simulink model "PV1000_STM32_767_ZI_state_control"  (R2023a)
settings: Solver=FixedStepAuto  StartTime=0.0  StopTime=inf  FixedStep=0.001  RelTol=1e-3
undefined symbols (not defined in the file): DiscIntNeverNeededParam
libraries: mbedblockslib x17, simulink x14, slpidlib x3, stmnucleolib x2, nucleoutilitieslib x1, etargetslib x1, dspswit3 x1
(part 1 of 2)
settings Model: SimulationMode=external  ExtModeTrigDuration=10  Creator=The MathWorks, Inc.  LastModifiedBy=roehren
settings SolverCC: AlgebraicLoopSolver=TrustRegion  AutoInsertRateTranBlk=on  MaxZcPerStep=1
settings DataIOCC: ReturnWorkspaceOutputs=off
settings OptimizationCC: DefaultParameterBehavior=Inlined  GainParamInheritBuiltInType=on  UseFloatMulNetSlope=on  DefaultUnderspecifiedDataType=single  UseSpecifiedMinMax=on  InlineInvariantSignals=on  ReuseModelBlockBuffer=off  PassReuseOutputArgsAs=Individual arguments  ZeroExternalMemoryAtStartup=off  ZeroInternalMemoryAtStartup=off  NoFixptDivByZeroProtection=on  EfficientFloat2IntCast=on  MaxStackSize=64  OptimizeBlockOrder=speed  EfficientTunableParamExpr=on
settings DebuggingCC: MultiTaskRateTransMsg=warning  ParameterTunabilityLossMsg=error  UnconnectedInputMsg=warning  UnconnectedOutputMsg=warning  UnconnectedLineMsg=warning  ArithmeticOperatorsInVariantConditions=warning
settings HardwareCC: ProdBitPerPointer=32  ProdBitPerSizeT=32  ProdBitPerPtrDiffT=32  ProdLargestAtomicInteger=Long  ProdLargestAtomicFloat=Double  ProdWordSize=32  ProdLongLongMode=on  ProdHWDeviceType=ARM Compatible->ARM Cortex
settings ModelReferenceCC: EnableRefExpFcnMdlSchedulingChecks=on
settings SFSimCC: SimUseLocalCustomCode=off  MATLABDynamicMemAlloc=off
settings RTWCC: Description=Embedded Coder  SystemTargetFile=ert.tlc  HardwareBoard=STM32 Nucleo F767ZI  TemplateMakefile=ert_default_tmf  GenerateReport=on  RTWUseLocalCustomCode=off  Toolchain=GNU Tools for ARM Embedded Processors  BuildConfiguration=Faster Runs  LaunchReport=on  DLArmComputeVersion=19.05
settings CodeAppCC: ForceParamTrailComments=on  OperatorAnnotations=on  StateflowObjectComments=on  MATLABSourceComments=on
settings ERTTargetCC: CodeReplacementLibrary=ARM Cortex-M (Optimized)  MultiwordLength=2048  CombineSignalStateStructs=on  ERTCustomFileBanners=off  SupportNonFinite=off  SupportContinuousTime=on  RemoveResetFunc=off  ModelStepFunctionPrototypeControlCompliant=off  ExtModeTransport=3  ExtModeStaticAlloc=on  ExtModeStaticAllocSize=2000  ExtModeMexFile=ext_xcp  ExtModeIntrfLevel=Level2 - Open
settings ConfigComp: CovMetricSettings=dsw  CovSaveCumulativeToWorkspaceVar=on  CovSaveSingleToWorkspaceVar=on  CovExternalEMLEnable=off

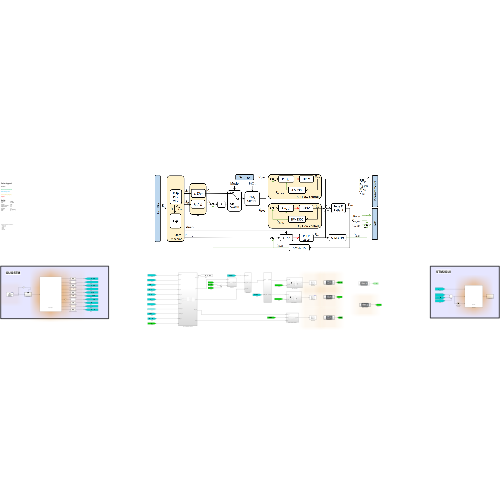
[thumbnail: Simulink's stored preview of the top-level diagram]
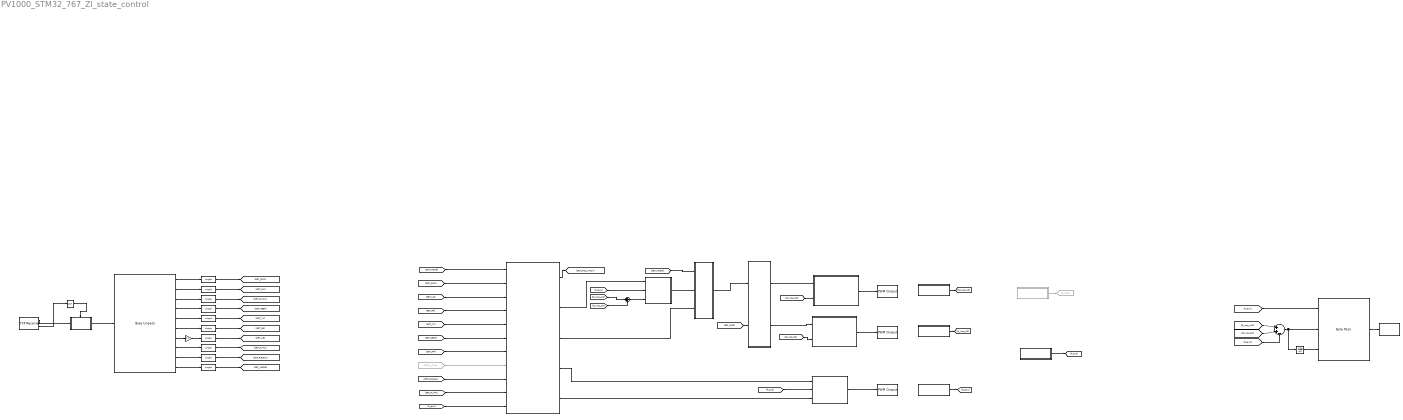
== system PV1000_STM32_767_ZI_state_control ==
  note: GUI2STM
  note: STM2GUI
  note: Color legend
      |
      | Boolean
      |
      | Sensor measurement
      |
      | Value set by user
      |
      | Event (rising edges)
      |
      | Output
      |
      | Units :
      | Pressure mbar
      | Flow L / min
      | Volume mL
      | Oxygen content %
      | Temperature °C
      | Humidity %
      | PWM 0...1 [a.u.]
      | Time s
  note: Mode Enum as defined in model InitFcn:
      | 0 BiPAP (t.b.a)
      | 1 CPAP (t.b.a)
      | 2 SPCV
      | 3 SVCV
      | 4 Standby
  "AMS 6915, I2C Bus 4" : Subsystem  Commented=on  TreatAsAtomicUnit=on  SystemSampleTime=0.05
  "AMS6915, I2C Bus 2" : Subsystem  TreatAsAtomicUnit=on  SystemSampleTime=0.01
  Byte Pack3 : nucleoutilitieslib/Byte Pack  datatypes={'single', 'single', 'single'}  byteAlign=1  blockPlatform=nucleo
  Byte Unpack1 : etargetslib/Byte Unpack  dimensions={[1], [1],[1], [1],[1], [1],[1], [1],[1], [1]}  datatypes={'uint8','uint8','uint8','uint8','uint16','uint8','uint8','uint8','uint8','uint8'}  byteAlign=1
  Data Type Conversion{1..10} (10 alike) : DataTypeConversion  OutDataTypeStr=single  SaturateOnIntegerOverflow=off  RndMeth=Floor
  Data Type Conversion11 : DataTypeConversion  Commented=on  OutDataTypeStr=single  SaturateOnIntegerOverflow=off  RndMeth=Floor
  Discrete-Time Integrator : DiscreteIntegrator  SampleTime=-1  ICPrevOutput=DiscIntNeverNeededParam  ICPrevScaledInput=DiscIntNeverNeededParam
  FiO2 Feedforward : Subsystem
  Flow_control_AIR : Subsystem
  Flow_control_O2 : Subsystem
  From18 : From  Commented=on  GotoTag=SET_F_Trig
  Gain : Gain  Gain=0.1
  Goto17 : Goto  Commented=on  GotoTag=P_insp
  NOT : Logic  Operator=NOT  IconShape=distinctive  AllPortsSameDT=off  OutDataTypeStr=boolean
  PEEP_threshold_detection : Subsystem
  PWM Output2 : mbedblockslib/PWM Output  Pin=PE_9  EnableInputFrequency=off  InitialFrequency=800  InitialDutyCycle=0  NotificationType=None
  PWM Output3 : mbedblockslib/PWM Output  Pin=PE_11  EnableInputFrequency=off  InitialFrequency=800  InitialDutyCycle=0  NotificationType=None
  PWM Output4 : mbedblockslib/PWM Output  Pin=PC_6  EnableInputFrequency=off  InitialFrequency=800  InitialDutyCycle=0  NotificationType=None
  "SFM3019, I2C Bus 4" : Subsystem  TreatAsAtomicUnit=on  SystemSampleTime=0.01
  "SFM3300, I2C Bus 2" : Subsystem  TreatAsAtomicUnit=on  SystemSampleTime=0.01
  "SFM3300, I2C Bus 4" : Subsystem  TreatAsAtomicUnit=on  SystemSampleTime=0.01
  State_and_Reference_Trajectory : Subsystem
  Subsystem : Subsystem  TreatAsAtomicUnit=on  SystemSampleTime=0.02
  Subsystem1 : Subsystem
  Subsystem3 : Subsystem
  Sum : Sum  Inputs=|++-
  Sum1 : Sum  Inputs=|++
  Swtich Mode : Subsystem
  TCP Receive3 : stmnucleolib/TCP Receive  Direction=Receive  ConnectionMode=Server  RemoteIPAddress=192.168.1.20  LocalPort=25005  ServerIPPort=25002  ByteOrder=BigEndian  BlockingMode=off  BlockTimeout=0.1  DataType=uint8  DataLength=11  OutputStatus=on  SampleTime=0.5
  wires:
  NOT/1 -> Subsystem3/Enable
  Subsystem3/1(Out1) -> Byte Unpack1/1
  Byte Unpack1/10 -> Data Type Conversion10/1
  Byte Unpack1/7 -> Gain/1
  TCP Receive3/1 -> Subsystem3/1(In1)
  Byte Unpack1/6 -> Data Type Conversion6/1
  Byte Unpack1/4 -> Data Type Conversion4/1
  TCP Receive3/2 -> NOT/1
  Byte Unpack1/5 -> Data Type Conversion5/1
  Byte Unpack1/3 -> Data Type Conversion3/1
  Byte Unpack1/9 -> Data Type Conversion9/1
  Byte Unpack1/1 -> Data Type Conversion1/1
  Byte Unpack1/2 -> Data Type Conversion2/1
  Byte Pack3/1 -> Subsystem/1(In1)
  Byte Unpack1/8 -> Data Type Conversion8/1
  "SFM3300, I2C Bus 2"/1(Output) -> [Q_insp_O2]
  "SFM3300, I2C Bus 4"/1(Output) -> [Q_insp_AIR]
  Sum/1 -> Discrete-Time Integrator/1, Byte Pack3/2
  [Q_insp_AIR] -> Sum/1
  [Q_exp] -> Sum/3
  "SFM3019, I2C Bus 4"/1(Output2) -> [Q_exp]
  "AMS 6915, I2C Bus 4"/1(Output3) -> Goto17/1
  [P_exp] -> Byte Pack3/1
  [Q_insp_O2] -> Sum/2
  Discrete-Time Integrator/1 -> Byte Pack3/3
  State_and_Reference_Trajectory/2(P_ref) -> Subsystem1/1(P_ref)
  [P_exp] -> Subsystem1/2(P_meas)
  Sum1/1 -> Subsystem1/3(In6)
  "AMS6915, I2C Bus 2"/1(Pressure [mbar]) -> [P_exp]
  Flow_control_AIR/1(Out1) -> PWM Output2/1
  [Q_insp_AIR] -> Sum1/1
  [Q_insp_O2] -> Sum1/2
  [SET_MODE] -> Swtich Mode/1(SET_MODE)
  Subsystem1/1(Q_ref_PCV) -> Swtich Mode/2(Q_ref_PCV)
  State_and_Reference_Trajectory/3(Q_ref) -> Swtich Mode/3(Q_ref_VCV)
  FiO2 Feedforward/1(Q_ref_AIR) -> Flow_control_AIR/1(Q_ref_AIR)
  FiO2 Feedforward/2(Q_ref_O2) -> Flow_control_O2/1(Q_ref_O2)
  Flow_control_O2/1(Out1) -> PWM Output3/1
  PEEP_threshold_detection/1(peep_pwm) -> PWM Output4/1
  State_and_Reference_Trajectory/4(PEEP_ref) -> PEEP_threshold_detection/1(PEEP_ref)
  [P_exp] -> PEEP_threshold_detection/2(PEEP_m)
  Data Type Conversion1/1 -> [SET_FIO2]
  Data Type Conversion2/1 -> [SET_PIP]
  Data Type Conversion3/1 -> [SET_P_MAX]
  Data Type Conversion4/1 -> [SET_PEEP]
  Data Type Conversion5/1 -> [SET_TV]
  Data Type Conversion6/1 -> [SET_RR]
  Data Type Conversion7/1 -> [SET_I_E]
  Data Type Conversion8/1 -> [SET_F_Trig]
  Data Type Conversion9/1 -> [SET_Plateau]
  Data Type Conversion10/1 -> [SET_MODE]
  Gain/1 -> Data Type Conversion7/1
  [SET_MODE] -> State_and_Reference_Trajectory/1(Mode_set)
  [SET_FIO2] -> State_and_Reference_Trajectory/2(O2_set)
  [SET_I_E] -> State_and_Reference_Trajectory/3(IE_set)
  [SET_RR] -> State_and_Reference_Trajectory/4(Freq_set)
  [SET_TV] -> State_and_Reference_Trajectory/5(VTidal_set)
  [SET_PEEP] -> State_and_Reference_Trajectory/6(PEEP_set)
  [SET_PIP] -> State_and_Reference_Trajectory/7(PInsp_set)
  From18/1 -> State_and_Reference_Trajectory/8(FInspTrig_set)
  [SET_Plateau] -> State_and_Reference_Trajectory/9(InspPause_set)
  [SET_P_MAX] -> State_and_Reference_Trajectory/10(PMax_set)
  [Q_insp_AIR] -> Flow_control_AIR/2(Q_m_AIR)
  [Q_insp_O2] -> Flow_control_O2/2(Q_m_O2)
  [P_exp] -> State_and_Reference_Trajectory/11(In11)
  State_and_Reference_Trajectory/1(FiO2) -> [SET_FIO2_Intern]
  State_and_Reference_Trajectory/5(isInsp) -> PEEP_threshold_detection/3(isInsp)
  Swtich Mode/1(Q_ref) -> FiO2 Feedforward/1(Q_ref)
  [SET_FIO2] -> FiO2 Feedforward/2(SET_FiO2)

== system PV1000_STM32_767_ZI_state_control/AMS 6915, I2C Bus 4 ==
  note: Measure pressure
  note: Data readout
  note: - No configuration required
      | - Pressure Sensor's I2C address: 0x28
  note: Read Data from Pressure Sensor
  AMS6915_calculate pressure3 : MATLAB Function  TreatAsAtomicUnit=on
  AMS6915_calculate_temperature3 : MATLAB Function  Commented=on  TreatAsAtomicUnit=on
  Goto18 : Goto  Commented=on  GotoTag=T_AMS6915_dC_II
  I2C Master Read3 : mbedblockslib/I2C Controller Read  I2CModule=4  Mode=Master  SlaveAddress=hex2dec('28')  SlaveByteOrder=BigEndian  Direction=Receiver  RegisterAddressMode=off  RegisterAddress=0  SlaveDataType=uint8  DataLength=4  NoAck=off  RepeatedStart=off  OutputStatus=off  SampleTime=-1
  Output3 : Outport
  wires:
  AMS6915_calculate pressure3/1(p) -> Output3/1
  AMS6915_calculate_temperature3/1(T) -> Goto18/1
  I2C Master Read3/1 -> AMS6915_calculate pressure3/1(digoutp), AMS6915_calculate_temperature3/1(digoutT)  "I2CRead"

== system PV1000_STM32_767_ZI_state_control/AMS6915, I2C Bus 2 ==
  note: - No configuration required
      | - Pressure Sensor's I2C address: 0x28
  note: Data readout
  note: Measure pressure
  note: Read Data from Pressure Sensor
  AMS6915_calculate pressure2 : MATLAB Function  TreatAsAtomicUnit=on
  AMS6915_calculate_temperature2 : MATLAB Function  Commented=on  TreatAsAtomicUnit=on
  I2C Master Read2 : mbedblockslib/I2C Controller Read  I2CModule=2  Mode=Master  SlaveAddress=hex2dec('28')  SlaveByteOrder=BigEndian  Direction=Receiver  RegisterAddressMode=off  RegisterAddress=0  SlaveDataType=uint8  DataLength=4  NoAck=off  RepeatedStart=off  OutputStatus=off  SampleTime=-1
  Terminator : Terminator  Commented=on
  Pressure [mbar] : Outport
  wires:
  AMS6915_calculate_temperature2/1(T) -> Terminator/1
  AMS6915_calculate pressure2/1(p) -> Pressure [mbar]/1
  I2C Master Read2/1 -> AMS6915_calculate_temperature2/1(digoutT), AMS6915_calculate pressure2/1(digoutp)  "I2CRead"

== system PV1000_STM32_767_ZI_state_control/FiO2 Feedforward ==
  Q_ref : Inport
  SET_FiO2 : Inport  Port=2
  CalcFInspO2_ref : Fcn  Expr=(u(1)-0.21)/0.79
  Fcn1 : Fcn  Expr=1-u(1)
  Gain1 : Gain  Gain=0.01
  Product : Product
  Product1 : Product
  Saturation1 : Saturate  UpperLimit=100  LowerLimit=21
  Q_ref_AIR : Outport  VectorParamsAs1DForOutWhenUnconnected=off
  Q_ref_O2 : Outport  Port=2  VectorParamsAs1DForOutWhenUnconnected=off
  wires:
  Q_ref/1 -> Product/2, Product1/2
  Fcn1/1 -> Product/1
  Product1/1 -> Q_ref_O2/1
  Product/1 -> Q_ref_AIR/1
  CalcFInspO2_ref/1 -> Fcn1/1, Product1/1
  SET_FiO2/1 -> Saturation1/1
  Gain1/1 -> CalcFInspO2_ref/1
  Saturation1/1 -> Gain1/1

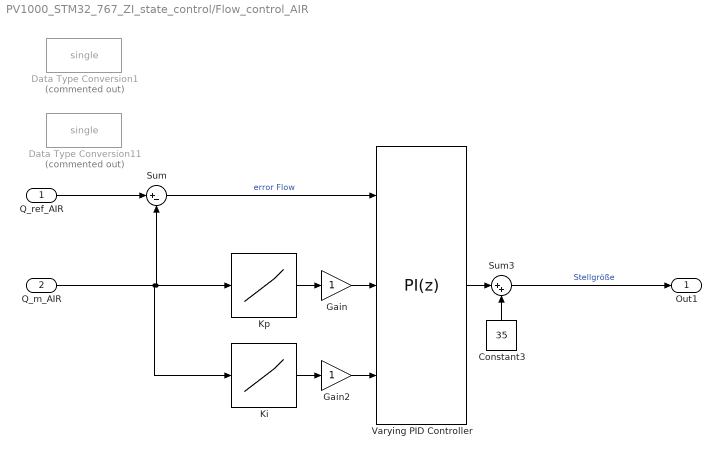
== system PV1000_STM32_767_ZI_state_control/Flow_control_AIR ==
  Q_ref_AIR : Inport
  Q_m_AIR : Inport  Port=2
  Constant3 : Constant  Value=35  OutDataTypeStr=double
  Data Type Conversion1 : DataTypeConversion  Commented=on  OutDataTypeStr=single  SaturateOnIntegerOverflow=off  RndMeth=Floor
  Data Type Conversion11 : DataTypeConversion  Commented=on  OutDataTypeStr=single  SaturateOnIntegerOverflow=off  RndMeth=Floor
  Gain : Gain
  Gain2 : Gain
  Ki : Lookup_n-D  NumberOfTableDimensions=1  BreakpointsForDimension1=[6 20 35 50]  Table=[26.4706 26.4706 26.4706 15.4412]  ExtrapMethod=Clip  InternalRulePriority=Speed  RndMeth=Simplest
  Kp : Lookup_n-D  NumberOfTableDimensions=1  BreakpointsForDimension1=[6 20 35 50]  Table=[0.2925 0.27 0.2475 0.1575]  ExtrapMethod=Clip  InternalRulePriority=Speed  RndMeth=Simplest
  Sum : Sum  Inputs=|+-
  Sum3 : Sum  Inputs=|++  AccumDataTypeStr=single
  Varying PID Controller : slpidlib/PID Controller  Controller=PI  Form=Parallel  TimeDomain=Discrete-time  UseExternalTs=off  SampleTime=-1  IntegratorMethod=Forward Euler  FilterMethod=Forward Euler  ControllerParametersSource=external  P=1  I=1  UseKiTs=off  D=0  N=100  UseFilter=on  TunerSelectOption=Transfer Function Based (PID Tuner App)  InitialConditionSource=internal  InitialConditionForIntegrator=0  InitialConditionForFilter=0  DifferentiatorICPrevScaledInput=0  ExternalReset=none  TrackingMode=off  Kt=1  LimitOutput=on  SatLimitsSource=internal  UpperSaturationLimit=60  LowerSaturationLimit=0  LinearizeAsGain=on  AntiWindupMode=clamping  Kb=1  LimitIntegrator=off  UpperIntegratorSaturationLimit=inf  LowerIntegratorSaturationLimit=-inf  PGainOutDataTypeStr=double  PProdOutDataTypeStr=double  POutMin=[]  POutMax=[]  IGainOutDataTypeStr=double  IProdOutDataTypeStr=double  IOutMin=[]  IOutMax=[]  DOutMin=[]  DOutMax=[]  NOutMin=[]  NOutMax=[]  SumOutDataTypeStr=double  SumOutMin=[]  SumOutMax=[]  SaturationOutDataTypeStr=double  SaturationOutMin=[]  SaturationOutMax=[]  PParamMin=[]  PParamMax=[]  IParamMin=[]  IParamMax=[]  DParamMin=[]  DParamMax=[]  NParamMin=[]  NParamMax=[]  KbParamMin=[]  KbParamMax=[]  KtParamMin=[]  KtParamMax=[]  KbOutMin=[]  KbOutMax=[]  KtOutMin=[]  KtOutMax=[]  IntegratorOutMin=[]  IntegratorOutMax=[]  FilterOutMin=[]  FilterOutMax=[]  SumI1OutMin=[]  SumI1OutMax=[]  SumI2OutMin=[]  SumI2OutMax=[]  SumI3OutMin=[]  SumI3OutMax=[]  SumI4OutMin=[]  SumI4OutMax=[]  SumDOutMin=[]  SumDOutMax=[]  SumAccumDataTypeStr=double  DifferentiatorOutMin=[]  DifferentiatorOutMax=[]  FilterDiffOutCoefMin=[]  FilterDiffOutCoefMax=[]  ReciprocalOutMin=[]  ReciprocalOutMax=[]  SumDenOutMin=[]  SumDenOutMax=[]  SumNumOutMin=[]  SumNumOutMax=[]  DivideOutMin=[]  DivideOutMax=[]  UdiffTsProdOutMin=[]  UdiffTsProdOutMax=[]  NTsProdOutMin=[]  NTsProdOutMax=[]  UintegralTsProdOutMin=[]  UintegralTsProdOutMax=[]  UngainTsProdOutMin=[]  UngainTsProdOutMax=[]  ClampingZeroOutDataTypeStr=Inherit: Inherit via back propagation  ClampingZeroOutMin=[]  ClampingZeroOutMax=[]  FilterDenConstantOutDataTypeStr=Inherit: Inherit via back propagation  FilterDenConstantOutMin=[]  FilterDenConstantOutMax=[]  PCopyOutDataTypeStr=Inherit: Inherit via back propagation  PCopyOutMin=[]  PCopyOutMax=[]  NCopyOutDataTypeStr=Inherit: Inherit via back propagation  NCopyOutMin=[]  NCopyOutMax=[]  IntegratorContinuousStateAttributes=''  IntegratorStateMustResolveToSignalObject=off  IntegratorRTWStateStorageClass=Auto  FilterContinuousStateAttributes=''  FilterStateMustResolveToSignalObject=off  FilterRTWStateStorageClass=Auto  ParallelPVariant=ExternalParameters  IdealPVariant=Disabled  IVariant=ExternalParameters  DVariant=Disabled  IntegratorVariant=Discrete  SatVariant=Enabled  AWVariant=DiscClampingParallel  PCopyVariant=Disabled  TRVariant=Disabled  FdbkBlocksVariant=Forward  IdealPFdbkVariant=Disabled  SatFdbkVariant=Disabled  DerivativeFilterVariant=Disabled  NVariant=Disabled  NCopyVariant=Disabled_SignalSpec  FilterICVariant=Disabled  IntegratorICVariant=InternalICs  ExternalResetVariant=Disabled  TRSumVariant=Passthrough  SumFdbkVariant=Disabled  SumVariant=Sum_PI  TsampFilterVariant=InternalTs  TsampNgainVariant=Passthrough  TsampIntegralVariant=Disabled_SignalSpec  ExternalSaturationOutDataTypeStr=Inherit: Same as second input
  Out1 : Outport
  wires:
  Gain2/1 -> Varying PID Controller/3
  Gain/1 -> Varying PID Controller/2
  Varying PID Controller/1 -> Sum3/1
  Sum3/1 -> Out1/1  "Stellgröße"
  Q_ref_AIR/1 -> Sum/1
  Sum/1 -> Varying PID Controller/1  "error Flow"
  Ki/1 -> Gain2/1
  Kp/1 -> Gain/1
  Constant3/1 -> Sum3/2
  Q_m_AIR/1 -> Sum/2, Kp/1, Ki/1

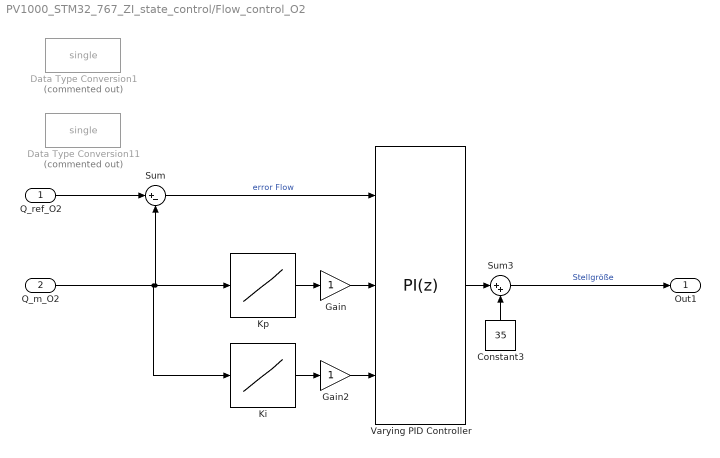
== system PV1000_STM32_767_ZI_state_control/Flow_control_O2 ==
  Q_ref_O2 : Inport
  Q_m_O2 : Inport  Port=2
  Constant3 : Constant  Value=35  OutDataTypeStr=double
  Data Type Conversion1 : DataTypeConversion  Commented=on  OutDataTypeStr=single  SaturateOnIntegerOverflow=off  RndMeth=Floor
  Data Type Conversion11 : DataTypeConversion  Commented=on  OutDataTypeStr=single  SaturateOnIntegerOverflow=off  RndMeth=Floor
  Gain : Gain
  Gain2 : Gain
  Ki : Lookup_n-D  NumberOfTableDimensions=1  BreakpointsForDimension1=[6 20 35 50]  Table=[26.4706 26.4706 26.4706 15.4412]  ExtrapMethod=Clip  InternalRulePriority=Speed  RndMeth=Simplest
  Kp : Lookup_n-D  NumberOfTableDimensions=1  BreakpointsForDimension1=[6 20 35 50]  Table=[0.2925 0.27 0.2475 0.1575]  ExtrapMethod=Clip  InternalRulePriority=Speed  RndMeth=Simplest
  Sum : Sum  Inputs=|+-
  Sum3 : Sum  Inputs=|++  AccumDataTypeStr=single
  Varying PID Controller : slpidlib/PID Controller  Controller=PI  Form=Parallel  TimeDomain=Discrete-time  UseExternalTs=off  SampleTime=-1  IntegratorMethod=Forward Euler  FilterMethod=Forward Euler  ControllerParametersSource=external  P=1  I=1  UseKiTs=off  D=0  N=100  UseFilter=on  TunerSelectOption=Transfer Function Based (PID Tuner App)  InitialConditionSource=internal  InitialConditionForIntegrator=0  InitialConditionForFilter=0  DifferentiatorICPrevScaledInput=0  ExternalReset=none  TrackingMode=off  Kt=1  LimitOutput=on  SatLimitsSource=internal  UpperSaturationLimit=60  LowerSaturationLimit=0  LinearizeAsGain=on  AntiWindupMode=clamping  Kb=1  LimitIntegrator=off  UpperIntegratorSaturationLimit=inf  LowerIntegratorSaturationLimit=-inf  PGainOutDataTypeStr=double  PProdOutDataTypeStr=double  POutMin=[]  POutMax=[]  IGainOutDataTypeStr=double  IProdOutDataTypeStr=double  IOutMin=[]  IOutMax=[]  DOutMin=[]  DOutMax=[]  NOutMin=[]  NOutMax=[]  SumOutDataTypeStr=double  SumOutMin=[]  SumOutMax=[]  SaturationOutDataTypeStr=double  SaturationOutMin=[]  SaturationOutMax=[]  PParamMin=[]  PParamMax=[]  IParamMin=[]  IParamMax=[]  DParamMin=[]  DParamMax=[]  NParamMin=[]  NParamMax=[]  KbParamMin=[]  KbParamMax=[]  KtParamMin=[]  KtParamMax=[]  KbOutMin=[]  KbOutMax=[]  KtOutMin=[]  KtOutMax=[]  IntegratorOutMin=[]  IntegratorOutMax=[]  FilterOutMin=[]  FilterOutMax=[]  SumI1OutMin=[]  SumI1OutMax=[]  SumI2OutMin=[]  SumI2OutMax=[]  SumI3OutMin=[]  SumI3OutMax=[]  SumI4OutMin=[]  SumI4OutMax=[]  SumDOutMin=[]  SumDOutMax=[]  SumAccumDataTypeStr=double  DifferentiatorOutMin=[]  DifferentiatorOutMax=[]  FilterDiffOutCoefMin=[]  FilterDiffOutCoefMax=[]  ReciprocalOutMin=[]  ReciprocalOutMax=[]  SumDenOutMin=[]  SumDenOutMax=[]  SumNumOutMin=[]  SumNumOutMax=[]  DivideOutMin=[]  DivideOutMax=[]  UdiffTsProdOutMin=[]  UdiffTsProdOutMax=[]  NTsProdOutMin=[]  NTsProdOutMax=[]  UintegralTsProdOutMin=[]  UintegralTsProdOutMax=[]  UngainTsProdOutMin=[]  UngainTsProdOutMax=[]  ClampingZeroOutDataTypeStr=Inherit: Inherit via back propagation  ClampingZeroOutMin=[]  ClampingZeroOutMax=[]  FilterDenConstantOutDataTypeStr=Inherit: Inherit via back propagation  FilterDenConstantOutMin=[]  FilterDenConstantOutMax=[]  PCopyOutDataTypeStr=Inherit: Inherit via back propagation  PCopyOutMin=[]  PCopyOutMax=[]  NCopyOutDataTypeStr=Inherit: Inherit via back propagation  NCopyOutMin=[]  NCopyOutMax=[]  IntegratorContinuousStateAttributes=''  IntegratorStateMustResolveToSignalObject=off  IntegratorRTWStateStorageClass=Auto  FilterContinuousStateAttributes=''  FilterStateMustResolveToSignalObject=off  FilterRTWStateStorageClass=Auto  ParallelPVariant=ExternalParameters  IdealPVariant=Disabled  IVariant=ExternalParameters  DVariant=Disabled  IntegratorVariant=Discrete  SatVariant=Enabled  AWVariant=DiscClampingParallel  PCopyVariant=Disabled  TRVariant=Disabled  FdbkBlocksVariant=Forward  IdealPFdbkVariant=Disabled  SatFdbkVariant=Disabled  DerivativeFilterVariant=Disabled  NVariant=Disabled  NCopyVariant=Disabled_SignalSpec  FilterICVariant=Disabled  IntegratorICVariant=InternalICs  ExternalResetVariant=Disabled  TRSumVariant=Passthrough  SumFdbkVariant=Disabled  SumVariant=Sum_PI  TsampFilterVariant=InternalTs  TsampNgainVariant=Passthrough  TsampIntegralVariant=Disabled_SignalSpec  ExternalSaturationOutDataTypeStr=Inherit: Same as second input
  Out1 : Outport
  wires:
  Q_m_O2/1 -> Ki/1, Kp/1, Sum/2
  Constant3/1 -> Sum3/2
  Kp/1 -> Gain/1
  Ki/1 -> Gain2/1
  Sum/1 -> Varying PID Controller/1  "error Flow"
  Q_ref_O2/1 -> Sum/1
  Sum3/1 -> Out1/1  "Stellgröße"
  Varying PID Controller/1 -> Sum3/1
  Gain/1 -> Varying PID Controller/2
  Gain2/1 -> Varying PID Controller/3

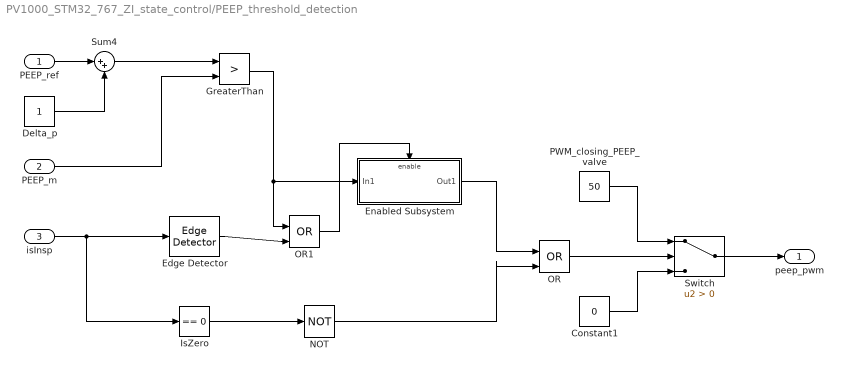
== system PV1000_STM32_767_ZI_state_control/PEEP_threshold_detection ==
  PEEP_ref : Inport
  PEEP_m : Inport  Port=2
  isInsp : Inport  Port=3
  Constant1 : Constant  Value=0  OutDataTypeStr=single
  Delta_p : Constant  OutDataTypeStr=single
  Edge Detector : dspswit3/Edge Detector  InputProcessing=Columns as channels (frame based)
  Enabled Subsystem : Subsystem  TreatAsAtomicUnit=on
  GreaterThan : RelationalOperator  Operator=>  OutDataTypeStr=boolean  RndMeth=Simplest  InputSameDT=off
  IsZero : simulink/Logic and Bit Operations/Compare To Zero  relop===  OutDataTypeStr=boolean
      settings: LibrarySourceBlock=|
      | simulink/Quick Insert/Logic and Bit
      | Operations/IsZero
  NOT : Logic  Operator=NOT  IconShape=distinctive  AllPortsSameDT=off  OutDataTypeStr=boolean
  OR : Logic  Operator=OR  IconShape=distinctive  AllPortsSameDT=off  OutDataTypeStr=boolean
  OR1 : Logic  Operator=OR  IconShape=distinctive  AllPortsSameDT=off  OutDataTypeStr=boolean
  PWM_closing_PEEP_valve : Constant  Value=50  OutDataTypeStr=single
  Sum4 : Sum  Inputs=|++
  Switch : Switch  Criteria=u2 > Threshold  SaturateOnIntegerOverflow=off  InputSameDT=off
  peep_pwm : Outport  OutDataTypeStr=single
  wires:
  OR1/1 -> Enabled Subsystem/Enable
  Edge Detector/1 -> OR1/2
  Enabled Subsystem/1(Out1) -> OR/1
  Sum4/1 -> GreaterThan/1
  Delta_p/1 -> Sum4/2
  GreaterThan/1 -> OR1/1, Enabled Subsystem/1(In1)
  OR/1 -> Switch/2
  NOT/1 -> OR/2
  Constant1/1 -> Switch/3
  PWM_closing_PEEP_valve/1 -> Switch/1
  Switch/1 -> peep_pwm/1
  IsZero/1 -> NOT/1
  PEEP_m/1 -> GreaterThan/2
  PEEP_ref/1 -> Sum4/1
  isInsp/1 -> IsZero/1, Edge Detector/1

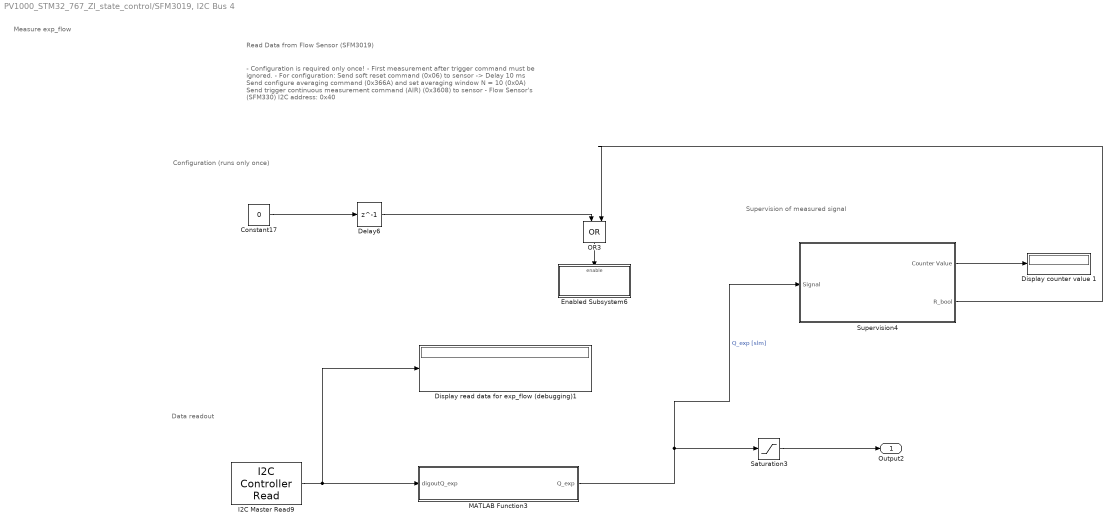
== system PV1000_STM32_767_ZI_state_control/SFM3019, I2C Bus 4 ==
  note: Measure exp_flow
  note: Configuration (runs only once)
  note: - Configuration is required only once!
      | - First measurement after trigger command must be ignored.
      | - For configuration:
      | Send soft reset command (0x06) to sensor -> Delay 10 ms
      | Send configure averaging command (0x366A) and set averaging window N = 10 (0x0A)
      | Send trigger continuous measurement command (AIR) (0x3608) to sensor
      | - Flow Sensor's (SFM330) I2C address: 0x40
  note: Read Data from Flow Sensor (SFM3019)
  note: Data readout
  note: Supervision of measured signal
  Constant17 : Constant  Value=0
  Delay6 : Delay  DelayLength=1  InitialCondition=1
  Display counter value 1 : Display
  Display read data for exp_flow (debugging)1 : Display
  Enabled Subsystem6 : Subsystem  TreatAsAtomicUnit=on
  I2C Master Read9 : mbedblockslib/I2C Controller Read  I2CModule=4  Mode=Master  SlaveAddress=hex2dec('2E')  SlaveByteOrder=BigEndian  Direction=Receiver  RegisterAddressMode=off  RegisterAddress=0  SlaveDataType=int8  DataLength=2  NoAck=off  RepeatedStart=off  OutputStatus=off  SampleTime=-1
  MATLAB Function3 : MATLAB Function  TreatAsAtomicUnit=on
  OR3 : Logic  Operator=OR  IconShape=distinctive  AllPortsSameDT=off  OutDataTypeStr=boolean
  Saturation3 : Saturate  UpperLimit=200  LowerLimit=0
  Supervision4 : Subsystem
  Output2 : Outport
  wires:
  Supervision4/2(R_bool) -> OR3/2
  I2C Master Read9/1 -> Display read data for exp_flow (debugging)1/1, MATLAB Function3/1(digoutQ_exp)
  Delay6/1 -> OR3/1
  Constant17/1 -> Delay6/1
  OR3/1 -> Enabled Subsystem6/Enable
  Supervision4/1(Counter Value) -> Display counter value 1/1
  MATLAB Function3/1(Q_exp) -> Saturation3/1, Supervision4/1(Signal)  "Q_exp [slm]"
  Saturation3/1 -> Output2/1

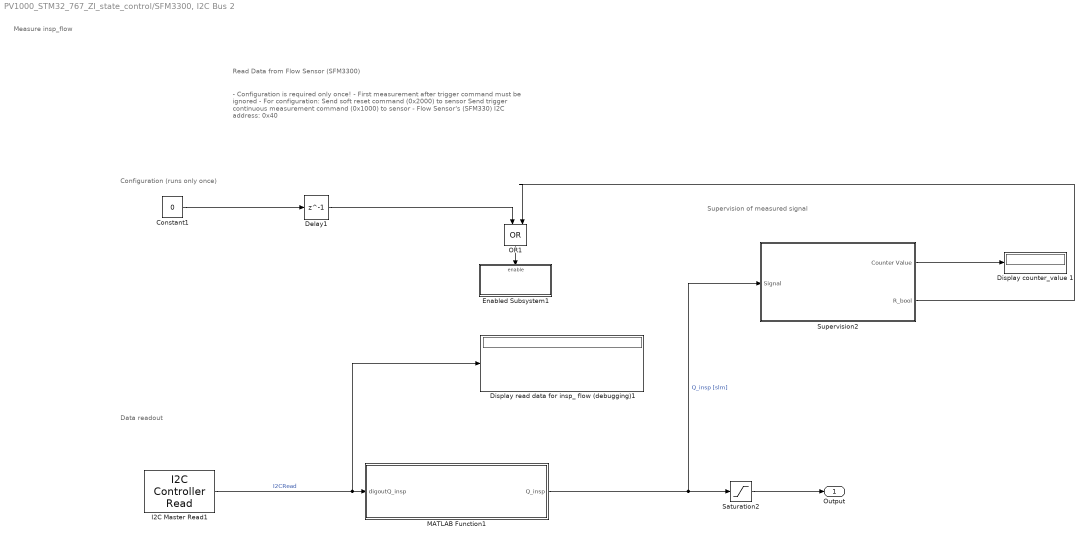
== system PV1000_STM32_767_ZI_state_control/SFM3300, I2C Bus 2 ==
  note: Supervision of measured signal
  note: Configuration (runs only once)
  note: Read Data from Flow Sensor (SFM3300)
  note: Data readout
  note: - Configuration is required only once!
      | - First measurement after trigger command must be ignored
      | - For configuration:
      | Send soft reset command (0x2000) to sensor
      | Send trigger continuous measurement command (0x1000) to sensor
      | - Flow Sensor's (SFM330) I2C address: 0x40
  note: Measure insp_flow
  Constant1 : Constant  Value=0
  Delay1 : Delay  DelayLength=1  InitialCondition=1
  Display counter_value 1 : Display
  Display read data for insp_ flow (debugging)1 : Display
  Enabled Subsystem1 : Subsystem  TreatAsAtomicUnit=on
  I2C Master Read1 : mbedblockslib/I2C Controller Read  I2CModule=2  Mode=Master  SlaveAddress=hex2dec('40')  SlaveByteOrder=BigEndian  Direction=Receiver  RegisterAddressMode=off  RegisterAddress=0  SlaveDataType=uint8  DataLength=3  NoAck=off  RepeatedStart=off  OutputStatus=off  SampleTime=-1
  MATLAB Function1 : MATLAB Function  TreatAsAtomicUnit=on
  OR1 : Logic  Operator=OR  IconShape=distinctive  AllPortsSameDT=off  OutDataTypeStr=boolean
  Saturation2 : Saturate  UpperLimit=200  LowerLimit=0
  Supervision2 : Subsystem
  Output : Outport
  wires:
  MATLAB Function1/1(Q_insp) -> Saturation2/1, Supervision2/1(Signal)  "Q_insp [slm]"
  OR1/1 -> Enabled Subsystem1/Enable
  Supervision2/2(R_bool) -> OR1/2
  Supervision2/1(Counter Value) -> Display counter_value 1/1
  Delay1/1 -> OR1/1
  I2C Master Read1/1 -> Display read data for insp_ flow (debugging)1/1, MATLAB Function1/1(digoutQ_insp)  "I2CRead"
  Constant1/1 -> Delay1/1
  Saturation2/1 -> Output/1

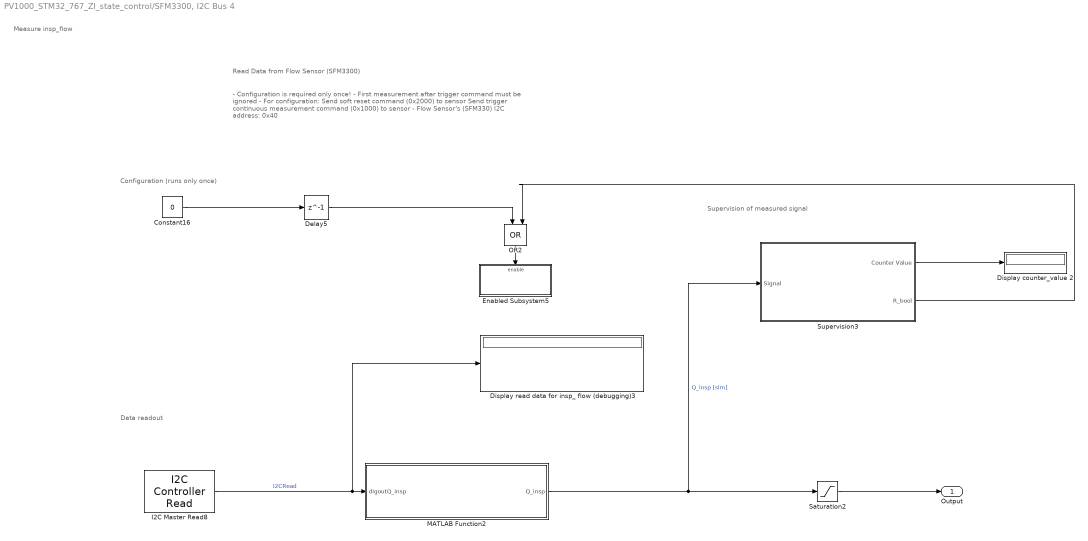
== system PV1000_STM32_767_ZI_state_control/SFM3300, I2C Bus 4 ==
  note: Data readout
  note: - Configuration is required only once!
      | - First measurement after trigger command must be ignored
      | - For configuration:
      | Send soft reset command (0x2000) to sensor
      | Send trigger continuous measurement command (0x1000) to sensor
      | - Flow Sensor's (SFM330) I2C address: 0x40
  note: Read Data from Flow Sensor (SFM3300)
  note: Supervision of measured signal
  note: Measure insp_flow
  note: Configuration (runs only once)
  Constant16 : Constant  Value=0
  Delay5 : Delay  DelayLength=1  InitialCondition=1
  Display counter_value 2 : Display
  Display read data for insp_ flow (debugging)3 : Display
  Enabled Subsystem5 : Subsystem  TreatAsAtomicUnit=on
  I2C Master Read8 : mbedblockslib/I2C Controller Read  I2CModule=4  Mode=Master  SlaveAddress=hex2dec('40')  SlaveByteOrder=BigEndian  Direction=Receiver  RegisterAddressMode=off  RegisterAddress=0  SlaveDataType=uint8  DataLength=3  NoAck=off  RepeatedStart=off  OutputStatus=off  SampleTime=-1
  MATLAB Function2 : MATLAB Function  TreatAsAtomicUnit=on
  OR2 : Logic  Operator=OR  IconShape=distinctive  AllPortsSameDT=off  OutDataTypeStr=boolean
  Saturation2 : Saturate  UpperLimit=200  LowerLimit=0
  Supervision3 : Subsystem
  Output : Outport
  wires:
  I2C Master Read8/1 -> Display read data for insp_ flow (debugging)3/1, MATLAB Function2/1(digoutQ_insp)  "I2CRead"
  Delay5/1 -> OR2/1
  Constant16/1 -> Delay5/1
  Supervision3/2(R_bool) -> OR2/2
  Supervision3/1(Counter Value) -> Display counter_value 2/1
  MATLAB Function2/1(Q_insp) -> Supervision3/1(Signal), Saturation2/1  "Q_insp [slm]"
  OR2/1 -> Enabled Subsystem5/Enable
  Saturation2/1 -> Output/1

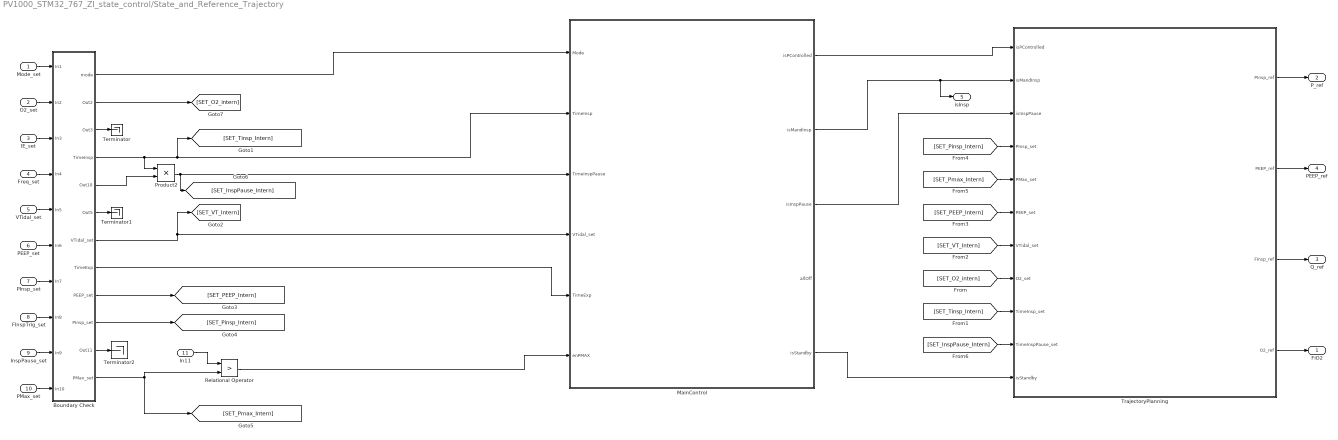
== system PV1000_STM32_767_ZI_state_control/State_and_Reference_Trajectory ==
  Mode_set : Inport
  O2_set : Inport  Port=2
  IE_set : Inport  Port=3
  Freq_set : Inport  Port=4
  VTidal_set : Inport  Port=5
  PEEP_set : Inport  Port=6
  PInsp_set : Inport  Port=7
  FInspTrig_set : Inport  Port=8
  InspPause_set : Inport  Port=9
  PMax_set : Inport  Port=10
  In11 : Inport  Port=11
  Boundary Check : Subsystem
  MainControl : Stateflow chart  TreatAsAtomicUnit=on
      settings: PortSchema="{\"entries\":[{\"content\":{\"sides\":[{\"content\":{\"connectorIds\":[\"In1\",\"In2\",\"In3\",\"In5\",\"In4\",\"In6\"]},\"type\":\"ConnectorPlacement.EquallySpacedRectSide\",\"uuid\":\"e30533d5-cda5-4606-a3d8-30b9129f327e\"},{\"content\":{\"connectorIds\":[\"Out1\",\"Out2\",\"Out3\",\"Out4\",\"Out5\"],\"side\":\"RIGHT\"},\"type\":\"ConnectorPlacement.EquallySpacedRectSide\",\"uuid\":\"5df88561-1b39-4d12-8c77-e629c1dade06\"},{\"content\":{\"side\":\"TOP\"},\"type\":\"ConnectorPlacement.EquallySpacedRectSide\",\"uuid\":\"c705e04d-f729-400f-a4a9-aee66c7b5de0\"}]},\"type\":\"ConnectorPlacement.EquallySpacedConnector\",\"uuid\":\"24d42db5-2501-402e-a152-1c17e1082f60\"}],\"packageUris\":[\"http://schema.mathworks.com/mf0/Connector/R2020b\"],\"version\":\"1.0\"}"
  Product2 : Product
  Relational Operator : RelationalOperator  Operator=>  OutDataTypeStr=boolean  RndMeth=Simplest  InputSameDT=off
  Terminator : Terminator
  Terminator1 : Terminator
  Terminator2 : Terminator
  TrajectoryPlanning : Stateflow chart  TreatAsAtomicUnit=on
      settings: PortSchema="{\"entries\":[{\"content\":{\"sides\":[{\"content\":{\"connectorIds\":[\"In2\",\"In3\",\"In4\",\"In5\",\"In6\",\"In7\",\"In8\",\"In9\",\"In10\",\"In11\",\"In1\"]},\"type\":\"ConnectorPlacement.EquallySpacedRectSide\",\"uuid\":\"9c8c731d-989c-4e85-a406-8b82eb5ceea0\"},{\"content\":{\"connectorIds\":[\"Out1\",\"Out2\",\"Out3\",\"Out4\"],\"side\":\"RIGHT\"},\"type\":\"ConnectorPlacement.EquallySpacedRectSide\",\"uuid\":\"fc0007b9-9033-48aa-b2dc-a6bede83aea2\"},{\"content\":{\"side\":\"TOP\"},\"type\":\"ConnectorPlacement.EquallySpacedRectSide\",\"uuid\":\"8a60c711-9e08-4968-a0b6-a904cd1439ba\"}]},\"type\":\"ConnectorPlacement.EquallySpacedConnector\",\"uuid\":\"4613fa66-4f5d-4ae5-8bab-ee2288b3867e\"}],\"packageUris\":[\"http://schema.mathworks.com/mf0/Connector/R2020b\"],\"version\":\"1.0\"}"
  FiO2 : Outport
  P_ref : Outport  Port=2
  Q_ref : Outport  Port=3
  PEEP_ref : Outport  Port=4
  isInsp : Outport  Port=5
  wires:
  Mode_set/1 -> Boundary Check/1(In1)
  O2_set/1 -> Boundary Check/2(In2)
  IE_set/1 -> Boundary Check/3(In3)
  Freq_set/1 -> Boundary Check/4(In4)
  VTidal_set/1 -> Boundary Check/5(In5)
  PEEP_set/1 -> Boundary Check/6(In6)
  PInsp_set/1 -> Boundary Check/7(In7)
  InspPause_set/1 -> Boundary Check/9(In9)
  FInspTrig_set/1 -> Boundary Check/8(In8)
  PMax_set/1 -> Boundary Check/10(In10)
  Boundary Check/1(mode) -> MainControl/1(Mode)
  Boundary Check/2(Out2) -> [SET_O2_intern]
  Boundary Check/3(Out3) -> Terminator/1
  Boundary Check/4(TimeInsp) -> MainControl/2(TimeInsp), [SET_Tinsp_Intern], Product2/1
  Boundary Check/6(Out5) -> Terminator1/1
  Boundary Check/7(VTidal_set) -> [SET_VT_Intern], MainControl/5(VTidal_set)
  Boundary Check/8(TimeExp) -> MainControl/4(TimeExp)
  Boundary Check/9(PEEP_set) -> [SET_PEEP_Intern]
  Boundary Check/10(PInsp_set) -> [SET_Pinsp_Intern]
  Boundary Check/5(Out10) -> Product2/2
  Boundary Check/11(Out11) -> Terminator2/1
  Boundary Check/12(PMax_set) -> Relational Operator/2, [SET_Pmax_Intern]
  Product2/1 -> [SET_InspPause_Intern], MainControl/3(TimeInspPause)
  TrajectoryPlanning/4(O2_ref) -> FiO2/1
  TrajectoryPlanning/3(FInsp_ref) -> Q_ref/1
  TrajectoryPlanning/2(PEEP_ref) -> PEEP_ref/1
  TrajectoryPlanning/1(PInsp_ref) -> P_ref/1
  In11/1 -> Relational Operator/1
  Relational Operator/1 -> MainControl/6(enPMAX)
  MainControl/1(isPControlled) -> TrajectoryPlanning/2(isPControlled)
  MainControl/5(isStandby) -> TrajectoryPlanning/1(isStandby)
  MainControl/3(isInspPause) -> TrajectoryPlanning/4(isInspPause)
  MainControl/2(isMandInsp) -> isInsp/1, TrajectoryPlanning/3(isMandInsp)
  [SET_O2_intern] -> TrajectoryPlanning/9(O2_set)
  [SET_Tinsp_Intern] -> TrajectoryPlanning/10(TimeInsp_set)
  [SET_VT_Intern] -> TrajectoryPlanning/8(VTidal_set)
  [SET_PEEP_Intern] -> TrajectoryPlanning/7(PEEP_set)
  [SET_Pinsp_Intern] -> TrajectoryPlanning/5(PInsp_set)
  [SET_Pmax_Intern] -> TrajectoryPlanning/6(PMax_set)
  [SET_InspPause_Intern] -> TrajectoryPlanning/11(TimeInspPause_set)

== system PV1000_STM32_767_ZI_state_control/Subsystem ==
  In1 : Inport
  TCP Send2 : stmnucleolib/TCP Send  Direction=Send  ConnectionMode=Server  RemoteIPAddress=192.168.1.20  LocalPort=25000  ServerIPPort=25000  ByteOrder=BigEndian  BlockingMode=off  BlockTimeout=0.1  DataType=uint8  DataLength=1  OutputStatus=off
  wires:
  In1/1 -> TCP Send2/1

== system PV1000_STM32_767_ZI_state_control/Subsystem1 ==
  P_ref : Inport
  P_meas : Inport  Port=2  OutDataTypeStr=single
  In6 : Inport  Port=3
  Data Type Conversion2 : DataTypeConversion  Commented=on  OutDataTypeStr=single  SaturateOnIntegerOverflow=off  RndMeth=Floor
  Gain1 : Gain  Gain=0.80
  PID Controller1 : slpidlib/PID Controller  Controller=P  Form=Parallel  TimeDomain=Discrete-time  UseExternalTs=off  SampleTime=-1  IntegratorMethod=Forward Euler  FilterMethod=Forward Euler  ControllerParametersSource=internal  P=0.5  I=1  UseKiTs=off  D=0  N=100  UseFilter=on  TunerSelectOption=Transfer Function Based (PID Tuner App)  InitialConditionSource=internal  InitialConditionForIntegrator=0  InitialConditionForFilter=0  DifferentiatorICPrevScaledInput=0  ExternalReset=none  TrackingMode=off  Kt=1  LimitOutput=off  SatLimitsSource=internal  UpperSaturationLimit=inf  LowerSaturationLimit=-inf  LinearizeAsGain=on  AntiWindupMode=none  Kb=1  LimitIntegrator=off  UpperIntegratorSaturationLimit=inf  LowerIntegratorSaturationLimit=-inf  POutMin=[]  POutMax=[]  IOutMin=[]  IOutMax=[]  DOutMin=[]  DOutMax=[]  NOutMin=[]  NOutMax=[]  SumOutMin=[]  SumOutMax=[]  SaturationOutMin=[]  SaturationOutMax=[]  PParamMin=[]  PParamMax=[]  IParamMin=[]  IParamMax=[]  DParamMin=[]  DParamMax=[]  NParamMin=[]  NParamMax=[]  KbParamMin=[]  KbParamMax=[]  KtParamMin=[]  KtParamMax=[]  KbOutMin=[]  KbOutMax=[]  KtOutMin=[]  KtOutMax=[]  IntegratorOutMin=[]  IntegratorOutMax=[]  FilterOutMin=[]  FilterOutMax=[]  SumI1OutMin=[]  SumI1OutMax=[]  SumI2OutMin=[]  SumI2OutMax=[]  SumI3OutMin=[]  SumI3OutMax=[]  SumI4OutMin=[]  SumI4OutMax=[]  SumDOutMin=[]  SumDOutMax=[]  DifferentiatorOutMin=[]  DifferentiatorOutMax=[]  FilterDiffOutCoefMin=[]  FilterDiffOutCoefMax=[]  ReciprocalOutMin=[]  ReciprocalOutMax=[]  SumDenOutMin=[]  SumDenOutMax=[]  SumNumOutMin=[]  SumNumOutMax=[]  DivideOutMin=[]  DivideOutMax=[]  UdiffTsProdOutMin=[]  UdiffTsProdOutMax=[]  NTsProdOutMin=[]  NTsProdOutMax=[]  UintegralTsProdOutMin=[]  UintegralTsProdOutMax=[]  UngainTsProdOutMin=[]  UngainTsProdOutMax=[]  ClampingZeroOutDataTypeStr=Inherit: Inherit via back propagation  ClampingZeroOutMin=[]  ClampingZeroOutMax=[]  FilterDenConstantOutDataTypeStr=Inherit: Inherit via back propagation  FilterDenConstantOutMin=[]  FilterDenConstantOutMax=[]  PCopyOutDataTypeStr=Inherit: Inherit via back propagation  PCopyOutMin=[]  PCopyOutMax=[]  NCopyOutDataTypeStr=Inherit: Inherit via back propagation  NCopyOutMin=[]  NCopyOutMax=[]  IntegratorContinuousStateAttributes=''  IntegratorStateMustResolveToSignalObject=off  IntegratorRTWStateStorageClass=Auto  FilterContinuousStateAttributes=''  FilterStateMustResolveToSignalObject=off  FilterRTWStateStorageClass=Auto  ParallelPVariant=InternalParameters  IdealPVariant=Disabled  IVariant=Disabled  DVariant=Disabled  IntegratorVariant=Disabled  SatVariant=Disabled  AWVariant=Disabled  PCopyVariant=Disabled  TRVariant=Disabled  FdbkBlocksVariant=Forward  IdealPFdbkVariant=Disabled  SatFdbkVariant=Disabled  DerivativeFilterVariant=Disabled  NVariant=Disabled  NCopyVariant=Disabled_SignalSpec  FilterICVariant=Disabled  IntegratorICVariant=Disabled  ExternalResetVariant=Disabled  TRSumVariant=Passthrough  SumFdbkVariant=Disabled  SumVariant=Passthrough_P  TsampFilterVariant=InternalTs  TsampNgainVariant=Passthrough  TsampIntegralVariant=Disabled_SignalSpec  ExternalSaturationOutDataTypeStr=Inherit: Same as second input
  Rate Transition4 : RateTransition
  Sum1 : Sum  Inputs=|+-
  Sum5 : Sum  Inputs=++|
  Q_ref_PCV : Outport
  wires:
  Sum5/1 -> Q_ref_PCV/1
  P_meas/1 -> Rate Transition4/1
  In6/1 -> Gain1/1
  PID Controller1/1 -> Sum5/2
  P_ref/1 -> Sum1/1
  Rate Transition4/1 -> Sum1/2
  Sum1/1 -> PID Controller1/1  "error Druck"
  Gain1/1 -> Sum5/1

== system PV1000_STM32_767_ZI_state_control/Subsystem3 ==
  In1 : Inport
  Enable : EnablePort
  Out1 : Outport
  wires:
  In1/1 -> Out1/1

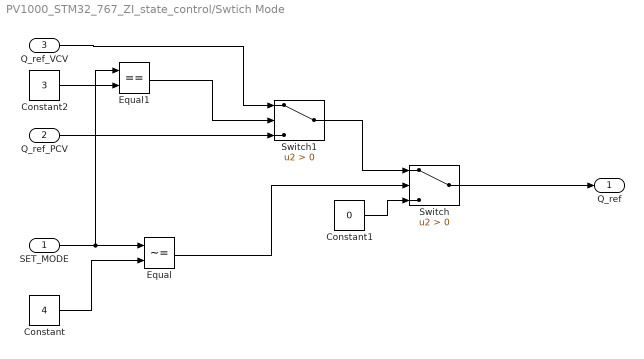
== system PV1000_STM32_767_ZI_state_control/Swtich Mode ==
  SET_MODE : Inport
  Q_ref_PCV : Inport  Port=2
  Q_ref_VCV : Inport  Port=3
  Constant : Constant  Value=4  OutDataTypeStr=single
  Constant1 : Constant  Value=0  OutDataTypeStr=single
  Constant2 : Constant  Value=3  OutDataTypeStr=single
  Equal : RelationalOperator  Operator=~=  OutDataTypeStr=boolean  RndMeth=Simplest  InputSameDT=off
  Equal1 : RelationalOperator  Operator===  OutDataTypeStr=boolean  RndMeth=Simplest  InputSameDT=off
  Switch : Switch  Criteria=u2 > Threshold  SaturateOnIntegerOverflow=off  InputSameDT=off
  Switch1 : Switch  Criteria=u2 > Threshold  SaturateOnIntegerOverflow=off  InputSameDT=off
  Q_ref : Outport
  wires:
  SET_MODE/1 -> Equal1/1, Equal/1
  Constant/1 -> Equal/2
  Equal/1 -> Switch/2
  Switch/1 -> Q_ref/1
  Constant2/1 -> Equal1/2
  Q_ref_VCV/1 -> Switch1/1
  Equal1/1 -> Switch1/2
  Q_ref_PCV/1 -> Switch1/3
  Switch1/1 -> Switch/1
  Constant1/1 -> Switch/3

== system PV1000_STM32_767_ZI_state_control/PEEP_threshold_detection/Enabled Subsystem ==
  In1 : Inport
  Enable : EnablePort
  Out1 : Outport
  wires:
  In1/1 -> Out1/1

== system PV1000_STM32_767_ZI_state_control/SFM3019, I2C Bus 4/Enabled Subsystem6 ==
  note: Configure the SFM019 sensor
  Enable : EnablePort
  "Configure Averaging command and set N = 10 " : Constant  Value=[hex2dec('36') hex2dec('6A') hex2dec('0A')]
  Data Type Conversion : DataTypeConversion  OutDataTypeStr=uint8  SaturateOnIntegerOverflow=off  RndMeth=Floor
  Data Type Conversion1 : DataTypeConversion  OutDataTypeStr=uint8  SaturateOnIntegerOverflow=off  RndMeth=Floor
  Data Type Conversion3 : DataTypeConversion  OutDataTypeStr=uint8  SaturateOnIntegerOverflow=off  RndMeth=Floor
  I2C Master Write : mbedblockslib/I2C Controller Write  I2CModule=4  Mode=Master  SlaveAddress=hex2dec('2E')  SlaveByteOrder=BigEndian  Direction=Transmitter  RegisterAddressMode=off  RegisterAddress=uint8(1)  SlaveDataType=uint8  DataLength=2  NoAck=off  RepeatedStart=off  OutputStatus=off
  I2C Master Write1 : mbedblockslib/I2C Controller Write  I2CModule=4  Mode=Master  SlaveAddress=hex2dec('2E')  SlaveByteOrder=BigEndian  Direction=Transmitter  RegisterAddressMode=off  RegisterAddress=uint8(1)  SlaveDataType=uint8  DataLength=2  NoAck=off  RepeatedStart=off  OutputStatus=off
  I2C Master Write2 : mbedblockslib/I2C Controller Write  I2CModule=4  Mode=Master  SlaveAddress=hex2dec('2E')  SlaveByteOrder=BigEndian  Direction=Transmitter  RegisterAddressMode=off  RegisterAddress=uint8(1)  SlaveDataType=uint8  DataLength=2  NoAck=off  RepeatedStart=off  OutputStatus=off
  "Soft rest command " : Constant  Value=[hex2dec('06')]
  Start continuous measurement command (AIR) : Constant  Value=[hex2dec('36') hex2dec('08')]
  wires:
  Start continuous measurement command (AIR)/1 -> Data Type Conversion3/1
  Data Type Conversion3/1 -> I2C Master Write/1
  Data Type Conversion1/1 -> I2C Master Write2/1
  "Configure Averaging command and set N = 10 "/1 -> Data Type Conversion1/1
  "Soft rest command "/1 -> Data Type Conversion/1
  Data Type Conversion/1 -> I2C Master Write1/1

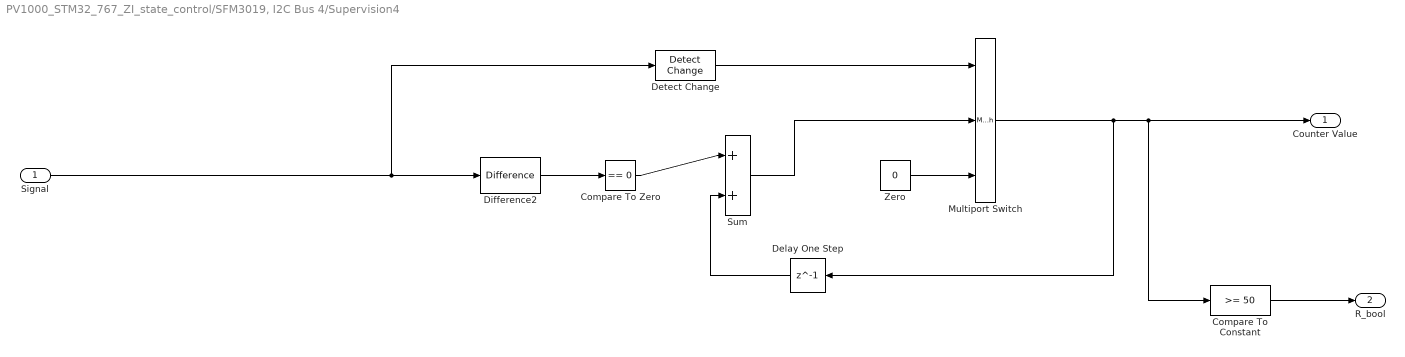
== system PV1000_STM32_767_ZI_state_control/SFM3019, I2C Bus 4/Supervision4 ==
  Signal : Inport
  Compare To Constant : simulink/Logic and Bit Operations/Compare To Constant  relop=>=  const=50  OutDataTypeStr=uint8
  Compare To Zero : simulink/Logic and Bit Operations/Compare To Zero  relop===  OutDataTypeStr=uint8
  Delay One Step : Delay  DelayLength=1
  Detect Change : simulink/Logic and Bit Operations/Detect Change  vinit=0  OutDataTypeStr=uint8
  Difference2 : simulink/Discrete/Difference  ICPrevInput=0.0  OutMin=[]  OutMax=[]  OutDataType=fixdt(1, 16)  OutScaling=2^-10  DoSatur=off
  Multiport Switch : MultiPortSwitch  DataPortOrder=Zero-based contiguous  Inputs=2  zeroidx=on  SaturateOnIntegerOverflow=off  InputSameDT=off
  Sum : Sum  Inputs=|++
  Zero : Constant  Value=0  OutDataTypeStr=Inherit: Inherit via back propagation
  Counter Value : Outport
  R_bool : Outport  Port=2
  wires:
  Compare To Constant/1 -> R_bool/1
  Zero/1 -> Multiport Switch/3
  Detect Change/1 -> Multiport Switch/1
  Multiport Switch/1 -> Counter Value/1, Compare To Constant/1, Delay One Step/1
  Delay One Step/1 -> Sum/2
  Difference2/1 -> Compare To Zero/1
  Sum/1 -> Multiport Switch/2
  Signal/1 -> Difference2/1, Detect Change/1
  Compare To Zero/1 -> Sum/1

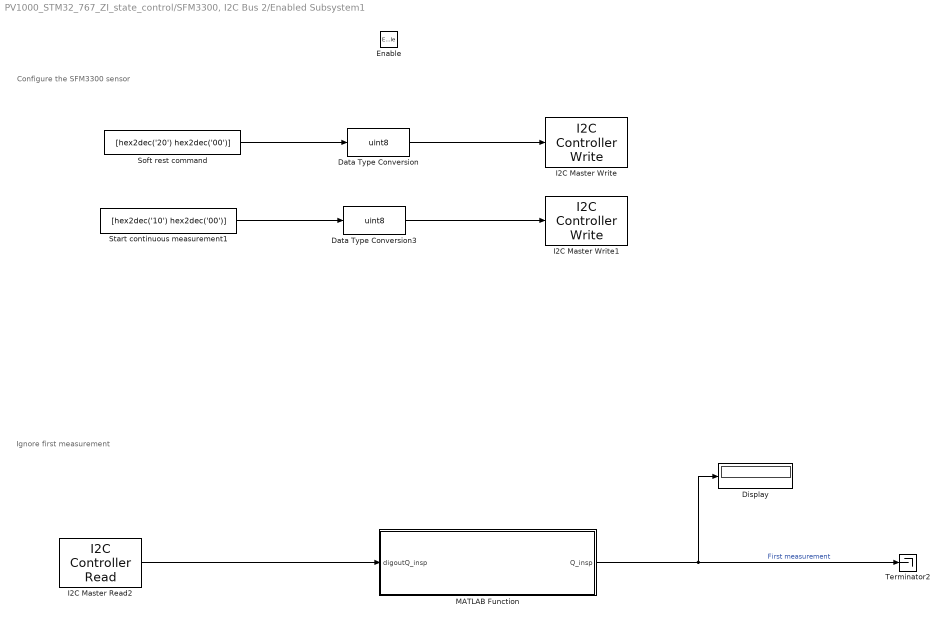
== system PV1000_STM32_767_ZI_state_control/SFM3300, I2C Bus 2/Enabled Subsystem1 ==
  note: Ignore first measurement
  note: Configure the SFM3300 sensor
  Enable : EnablePort
  Data Type Conversion : DataTypeConversion  OutDataTypeStr=uint8  SaturateOnIntegerOverflow=off  RndMeth=Floor
  Data Type Conversion3 : DataTypeConversion  OutDataTypeStr=uint8  SaturateOnIntegerOverflow=off  RndMeth=Floor
  Display : Display
  I2C Master Read2 : mbedblockslib/I2C Controller Read  I2CModule=2  Mode=Master  SlaveAddress=hex2dec('40')  SlaveByteOrder=BigEndian  Direction=Receiver  RegisterAddressMode=off  RegisterAddress=0  SlaveDataType=uint8  DataLength=3  NoAck=off  RepeatedStart=off  OutputStatus=off  SampleTime=-1
  I2C Master Write : mbedblockslib/I2C Controller Write  I2CModule=2  Mode=Master  SlaveAddress=hex2dec('40')  SlaveByteOrder=BigEndian  Direction=Transmitter  RegisterAddressMode=off  RegisterAddress=uint8(1)  SlaveDataType=uint8  DataLength=2  NoAck=off  RepeatedStart=off  OutputStatus=off
  I2C Master Write1 : mbedblockslib/I2C Controller Write  I2CModule=2  Mode=Master  SlaveAddress=hex2dec('40')  SlaveByteOrder=BigEndian  Direction=Transmitter  RegisterAddressMode=off  RegisterAddress=uint8(1)  SlaveDataType=uint8  DataLength=2  NoAck=off  RepeatedStart=off  OutputStatus=off
  MATLAB Function : MATLAB Function  TreatAsAtomicUnit=on
  "Soft rest command " : Constant  Value=[hex2dec('20') hex2dec('00')]
  Start continuous measurement1 : Constant  Value=[hex2dec('10') hex2dec('00')]
  Terminator2 : Terminator
  wires:
  Data Type Conversion/1 -> I2C Master Write/1
  "Soft rest command "/1 -> Data Type Conversion/1
  I2C Master Read2/1 -> MATLAB Function/1(digoutQ_insp)
  MATLAB Function/1(Q_insp) -> Terminator2/1, Display/1  "First measurement"
  Data Type Conversion3/1 -> I2C Master Write1/1
  Start continuous measurement1/1 -> Data Type Conversion3/1

== system PV1000_STM32_767_ZI_state_control/SFM3300, I2C Bus 2/Supervision2 ==
  Signal : Inport
  Compare To Constant : simulink/Logic and Bit Operations/Compare To Constant  relop=>=  const=50  OutDataTypeStr=uint8
  Compare To Zero : simulink/Logic and Bit Operations/Compare To Zero  relop===  OutDataTypeStr=uint8
  Delay One Step : Delay  DelayLength=1
  Detect Change : simulink/Logic and Bit Operations/Detect Change  vinit=0  OutDataTypeStr=uint8
  Difference2 : simulink/Discrete/Difference  ICPrevInput=0.0  OutMin=[]  OutMax=[]  OutDataType=fixdt(1, 16)  OutScaling=2^-10  DoSatur=off
  Multiport Switch : MultiPortSwitch  DataPortOrder=Zero-based contiguous  Inputs=2  zeroidx=on  SaturateOnIntegerOverflow=off  InputSameDT=off
  Sum : Sum  Inputs=|++
  Zero : Constant  Value=0  OutDataTypeStr=Inherit: Inherit via back propagation
  Counter Value : Outport
  R_bool : Outport  Port=2
  wires:
  Compare To Zero/1 -> Sum/1
  Signal/1 -> Detect Change/1, Difference2/1
  Sum/1 -> Multiport Switch/2
  Difference2/1 -> Compare To Zero/1
  Delay One Step/1 -> Sum/2
  Multiport Switch/1 -> Delay One Step/1, Compare To Constant/1, Counter Value/1
  Detect Change/1 -> Multiport Switch/1
  Zero/1 -> Multiport Switch/3
  Compare To Constant/1 -> R_bool/1

== system PV1000_STM32_767_ZI_state_control/SFM3300, I2C Bus 4/Enabled Subsystem5 ==
  note: Ignore first measurement
  note: Configure the SFM3300 sensor
  Enable : EnablePort
  Data Type Conversion : DataTypeConversion  OutDataTypeStr=uint8  SaturateOnIntegerOverflow=off  RndMeth=Floor
  Data Type Conversion3 : DataTypeConversion  OutDataTypeStr=uint8  SaturateOnIntegerOverflow=off  RndMeth=Floor
  Display : Display
  I2C Master Read8 : mbedblockslib/I2C Controller Read  I2CModule=4  Mode=Master  SlaveAddress=hex2dec('40')  SlaveByteOrder=BigEndian  Direction=Receiver  RegisterAddressMode=off  RegisterAddress=0  SlaveDataType=uint8  DataLength=3  NoAck=off  RepeatedStart=off  OutputStatus=off  SampleTime=-1
  I2C Master Write1 : mbedblockslib/I2C Controller Write  I2CModule=4  Mode=Master  SlaveAddress=hex2dec('40')  SlaveByteOrder=BigEndian  Direction=Transmitter  RegisterAddressMode=off  RegisterAddress=uint8(1)  SlaveDataType=uint8  DataLength=2  NoAck=off  RepeatedStart=off  OutputStatus=off
  I2C Master Write2 : mbedblockslib/I2C Controller Write  I2CModule=4  Mode=Master  SlaveAddress=hex2dec('40')  SlaveByteOrder=BigEndian  Direction=Transmitter  RegisterAddressMode=off  RegisterAddress=uint8(1)  SlaveDataType=uint8  DataLength=2  NoAck=off  RepeatedStart=off  OutputStatus=off
  MATLAB Function : MATLAB Function  TreatAsAtomicUnit=on
  "Soft rest command " : Constant  Value=[hex2dec('20') hex2dec('00')]
  Start continuous measurement1 : Constant  Value=[hex2dec('10') hex2dec('00')]
  Terminator2 : Terminator
  wires:
  Data Type Conversion/1 -> I2C Master Write2/1
  "Soft rest command "/1 -> Data Type Conversion/1
  I2C Master Read8/1 -> MATLAB Function/1(digoutQ_insp)
  MATLAB Function/1(Q_insp) -> Terminator2/1, Display/1  "First measurement"
  Data Type Conversion3/1 -> I2C Master Write1/1
  Start continuous measurement1/1 -> Data Type Conversion3/1

== system PV1000_STM32_767_ZI_state_control/SFM3300, I2C Bus 4/Supervision3 ==
  Signal : Inport
  Compare To Constant : simulink/Logic and Bit Operations/Compare To Constant  relop=>=  const=50  OutDataTypeStr=uint8
  Compare To Zero : simulink/Logic and Bit Operations/Compare To Zero  relop===  OutDataTypeStr=uint8
  Delay One Step : Delay  DelayLength=1
  Detect Change : simulink/Logic and Bit Operations/Detect Change  vinit=0  OutDataTypeStr=uint8
  Difference2 : simulink/Discrete/Difference  ICPrevInput=0.0  OutMin=[]  OutMax=[]  OutDataType=fixdt(1, 16)  OutScaling=2^-10  DoSatur=off
  Multiport Switch : MultiPortSwitch  DataPortOrder=Zero-based contiguous  Inputs=2  zeroidx=on  SaturateOnIntegerOverflow=off  InputSameDT=off
  Sum : Sum  Inputs=|++
  Zero : Constant  Value=0  OutDataTypeStr=Inherit: Inherit via back propagation
  Counter Value : Outport
  R_bool : Outport  Port=2
  wires:
  Compare To Zero/1 -> Sum/1
  Signal/1 -> Detect Change/1, Difference2/1
  Sum/1 -> Multiport Switch/2
  Difference2/1 -> Compare To Zero/1
  Delay One Step/1 -> Sum/2
  Multiport Switch/1 -> Delay One Step/1, Compare To Constant/1, Counter Value/1
  Detect Change/1 -> Multiport Switch/1
  Zero/1 -> Multiport Switch/3
  Compare To Constant/1 -> R_bool/1

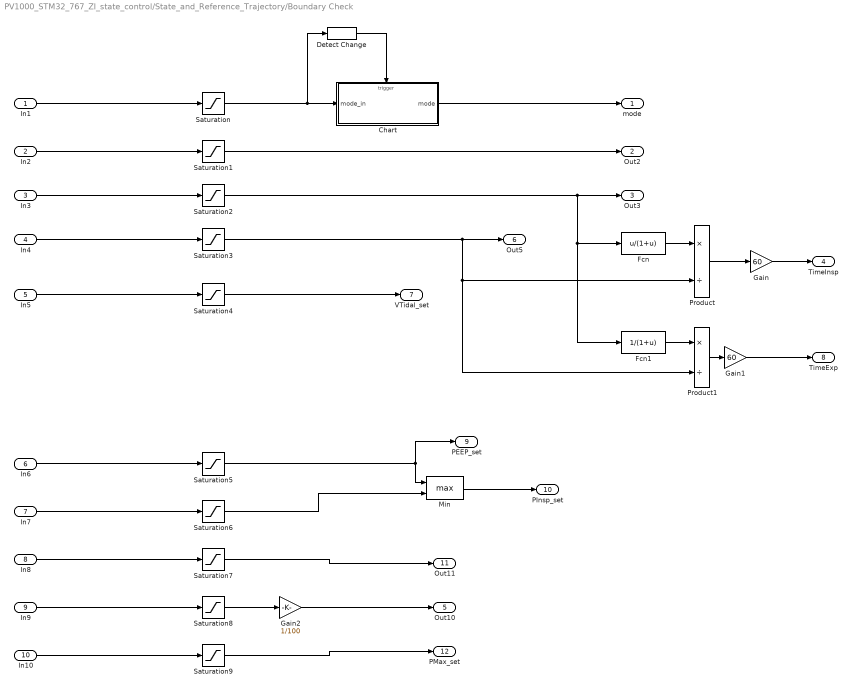
== system PV1000_STM32_767_ZI_state_control/State_and_Reference_Trajectory/Boundary Check ==
  In1 : Inport
  In2 : Inport  Port=2
  In3 : Inport  Port=3
  In4 : Inport  Port=4
  In5 : Inport  Port=5
  In6 : Inport  Port=6
  In7 : Inport  Port=7
  In8 : Inport  Port=8
  In9 : Inport  Port=9
  In10 : Inport  Port=10
  Chart : Stateflow chart  TreatAsAtomicUnit=on
  Detect Change : simulink/Logic and Bit Operations/Detect Change  vinit=100  OutDataTypeStr=boolean
  Fcn : Fcn  Expr=u/(1+u)
  Fcn1 : Fcn  Expr=1/(1+u)
  Gain : Gain  Gain=60
  Gain1 : Gain  Gain=60
  Gain2 : Gain  Gain=1/100
  Min : MinMax  Function=max  Inputs=2
  Product : Product  Inputs=*/
  Product1 : Product  Inputs=*/
  Saturation : Saturate  UpperLimit=5  LowerLimit=0
  Saturation1 : Saturate  UpperLimit=100  LowerLimit=20
  Saturation2 : Saturate  UpperLimit=4  LowerLimit=0.25
  Saturation{3,5..6,9} (4 alike) : Saturate  UpperLimit=60  LowerLimit=0
  Saturation4 : Saturate  UpperLimit=1000  LowerLimit=0
  Saturation7 : Saturate  UpperLimit=200  LowerLimit=0
  Saturation8 : Saturate  UpperLimit=50  LowerLimit=0
  mode : Outport
  Out2 : Outport  Port=2
  Out3 : Outport  Port=3
  TimeInsp : Outport  Port=4
  Out10 : Outport  Port=5
  Out5 : Outport  Port=6
  VTidal_set : Outport  Port=7
  TimeExp : Outport  Port=8
  PEEP_set : Outport  Port=9
  PInsp_set : Outport  Port=10
  Out11 : Outport  Port=11
  PMax_set : Outport  Port=12
  wires:
  In10/1 -> Saturation9/1
  Gain2/1 -> Out10/1
  Saturation2/1 -> Fcn1/1, Fcn/1, Out3/1
  Saturation8/1 -> Gain2/1
  Fcn1/1 -> Product1/1
  In8/1 -> Saturation7/1
  Saturation/1 -> Chart/1(mode_in), Detect Change/1
  Saturation3/1 -> Product/2, Product1/2, Out5/1
  Chart/1(mode) -> mode/1
  In5/1 -> Saturation4/1
  In7/1 -> Saturation6/1
  Saturation9/1 -> PMax_set/1
  In1/1 -> Saturation/1
  Saturation5/1 -> Min/1, PEEP_set/1
  Saturation6/1 -> Min/2
  Product1/1 -> Gain1/1
  In9/1 -> Saturation8/1
  Fcn/1 -> Product/1
  Product/1 -> Gain/1
  Detect Change/1 -> Chart/Trigger
  Gain1/1 -> TimeExp/1
  Saturation4/1 -> VTidal_set/1
  Gain/1 -> TimeInsp/1
  Min/1 -> PInsp_set/1
  In3/1 -> Saturation2/1
  Saturation7/1 -> Out11/1
  Saturation1/1 -> Out2/1
  In4/1 -> Saturation3/1
  In6/1 -> Saturation5/1
  In2/1 -> Saturation1/1
